simulink model "model1"  (R2014b)
settings: Solver=ode45  StartTime=0.0  StopTime=4.0  RelTol=1e-3
values from neighbouring files (symbols this model uses):
  A = [0 0 1 0;0 0 0 1;0 (r*(Mp^2)*(lp^2)*g)/(Jp*Jeq + Mp*(lp^2)*Jeq + Jp*Mp*(r^2)) -(Kt*Km)*(Jp+Mp*(lp^2))/((Jp*Jeq + Mp*(lp^2)*Jeq + Jp*Mp*(r^2))*(Rm)) 0;0 (Mp*lp*g*(Jeq + Mp*(r^2)))/(Jp*Jeq + Mp*(lp^2)*Jeq + Jp*Mp*(r^2)) -1*(Mp*lp*Kt*r*Km)/((Jp*Jeq + Mp*(lp^2)*Jeq + Jp*Mp*(r^2))*Rm) 0]    [invpendulum.m]
  B = [0;0;Kt*(Jp+Mp*(lp^2))/((Jp*Jeq + Mp*(lp^2)*Jeq + Jp*Mp*(r^2))*Rm);(Mp*lp*Kt*r)/((Jp*Jeq + Mp*(lp^2)*Jeq + Jp*Mp*(r^2))*Rm)]    [invpendulum.m]
  C = eye(4)    [invpendulum.m]
  D = zeros(4,1)    [invpendulum.m]
libraries: cstblocks x1, RCTblocks x1
settings Model: Creator=cclab  LastModifiedBy=cclab

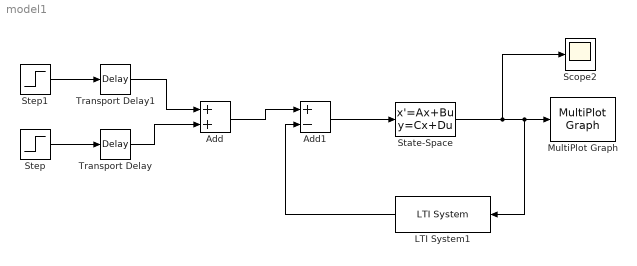
== system model1 ==
  Add : Sum
  Add1 : Sum  Inputs=+-
  LTI System1 : cstblocks/LTI System  sys=K  IC=[]
  MultiPlot Graph : RCTblocks/MultiPlot Graph  Tag=MultiPlot  tmin=0  tmax=5  ymin=-0.5  ymax=0.5  Tsamp=-1  titleString=Q=[1 1 1 1] R=[0.01]  vnamesave=multisimout
  Scope2 : Scope
  State-Space : StateSpace  A=A  B=B  C=C  D=D  X0=0
  Step : Step  Time=0.01  After=-3  SampleTime=0
  Step1 : Step  Time=0.01  After=3  SampleTime=0
  Transport Delay : TransportDelay  DelayTime=1.05
  Transport Delay1 : TransportDelay
  wires:
  Step/1 -> Transport Delay/1
  Transport Delay/1 -> Add/2
  Step1/1 -> Transport Delay1/1
  Transport Delay1/1 -> Add/1
  LTI System1/1 -> Add1/2
  Add1/1 -> State-Space/1
  State-Space/1 -> Scope2/1, LTI System1/1, MultiPlot Graph/1
  Add/1 -> Add1/1
